simulink model "MassDamper"  (R2024b)
settings: Solver=VariableStepAuto  StartTime=0.0  StopTime=10.0  RelTol=1e-3
settings Model: Creator=Seb  LastModifiedBy=Seb

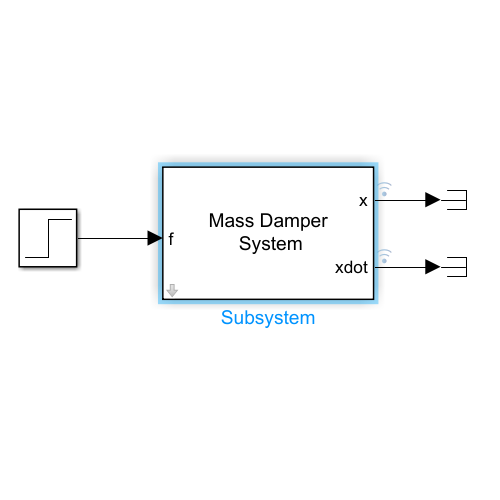
[thumbnail: Simulink's stored preview of the top-level diagram]
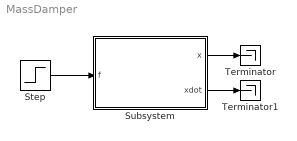
== system MassDamper ==
  Step : Step  After=1000  SampleTime=0
  Subsystem : Subsystem  mask{m=250, c=1000, k=10000}
      mask prompts: m "Mass"; c "Damping Rate"; k "Spring Stiffness"
      mask Display: fprintf("Mass Damper\n System")
  Terminator : Terminator
  Terminator1 : Terminator
  wires:
  Subsystem/1(x) -> Terminator/1
  Subsystem/2(xdot) -> Terminator1/1
  Step/1 -> Subsystem/1(f)

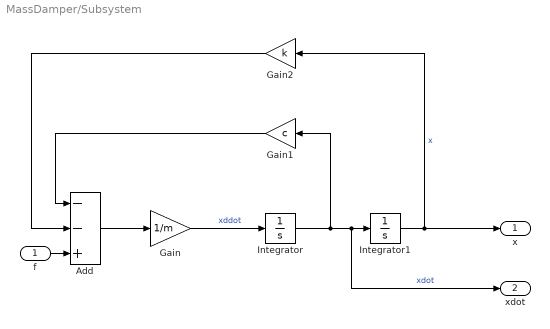
== system MassDamper/Subsystem ==
  f : Inport
  Add : Sum  Inputs=--+
  Gain : Gain  Gain=1/m
  Gain1 : Gain  Gain=c
  Gain2 : Gain  Gain=k
  Integrator : Integrator
  Integrator1 : Integrator
  x : Outport
  xdot : Outport  Port=2
  wires:
  Add/1 -> Gain/1
  Gain1/1 -> Add/1
  Gain2/1 -> Add/2
  Integrator1/1 -> x/1, Gain2/1  "x"
  f/1 -> Add/3
  Integrator/1 -> xdot/1, Integrator1/1, Gain1/1  "xdot"
  Gain/1 -> Integrator/1  "xddot"
